simulink model "Nov21_1"  (R2018b)
settings: Solver=VariableStepAuto  StartTime=0.0  StopTime=10.0  RelTol=1e-3
settings Model: Creator=Sandeep  LastModifiedBy=Sandeep

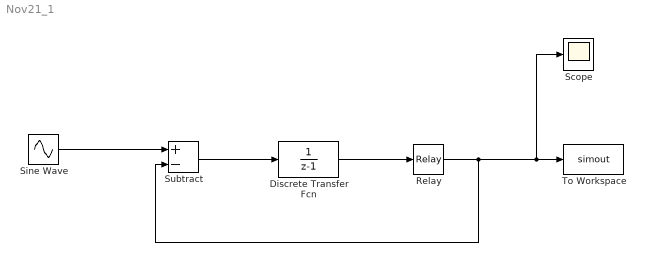
== system Nov21_1 ==
  Discrete Transfer Fcn : DiscreteTransferFcn  Denominator=[1 -1]  SampleTime=5e-8
  Relay : Relay  OnSwitchValue=0.5  OffSwitchValue=0.5
  Scope : Scope
  Sine Wave : Sin  Amplitude=0.2  Bias=0.5  Frequency=31.7e3  SampleTime=5e-8
  Subtract : Sum  Inputs=+-
  To Workspace : ToWorkspace  VariableName=simout  SaveFormat=Timeseries  SampleTime=-1
  wires:
  Sine Wave/1 -> Subtract/1
  Subtract/1 -> Discrete Transfer Fcn/1
  Discrete Transfer Fcn/1 -> Relay/1
  Relay/1 -> Subtract/2, Scope/1, To Workspace/1
